simulink model "olamodel"  (Simulink 8.3)
settings: Solver=FixedStepDiscrete  SolverMode=SingleTasking  StartTime=0.0  StopTime=9999999  RelTol=1e-3  AbsTol=1e-6
model workspace (MATLAB code in the model file):
  | olademo
values from neighbouring files (symbols this model uses):
  Fs = AR.SampleRate    [GenDSPTestbenchExample.m]    (also in HelperAircraftKalmanFilter.m = 1000; HelperAudioEqualization.m = 44100; HelperAudioEqualizationCodeGeneration.m = 44100; HelperAudioToneRemoval.m = 44100)
undefined symbols (not defined in the file or in its folder): bitrevorder, ymax, ymin
libraries: dspmathops x3, dspxfrm3 x2, dspsrcs4 x1, dspsigops x1, dspmisc x1, simulink x1
settings Model: Creator=The MathWorks Inc.  CovMetricSettings=d  ExtModeTrigMode=oneshot  ExtModeArmWhenConnect=off
settings DataIOCC: LimitDataPoints=off  SaveOutput=off  SaveTime=off  SignalLoggingName=logsOut
settings OptimizationCC: BlockReduction=off  BooleanDataType=off  ExpressionDepthLimit=2147483647  RollThreshold=2  InitFltsAndDblsToZero=on  EfficientMapNaN2IntZero=off
settings DebuggingCC: SaveWithParameterizedLinksMsg=none  SignalResolutionControl=TryResolveAllWithWarning  SolverPrmCheckMsg=none  MultiTaskDSMMsg=warning  MultiTaskCondExecSysMsg=none  IntegerOverflowMsg=none  FcnCallInpInsideContextMsg=UseLocalSettings  StrictBusMsg=None
settings HardwareCC: ProdHWDeviceType=Specified
settings RTWCC: IncludeERTFirstTime=on
settings GRTTargetCC: TargetFcnLib=ansi_tfl_tmw.mat

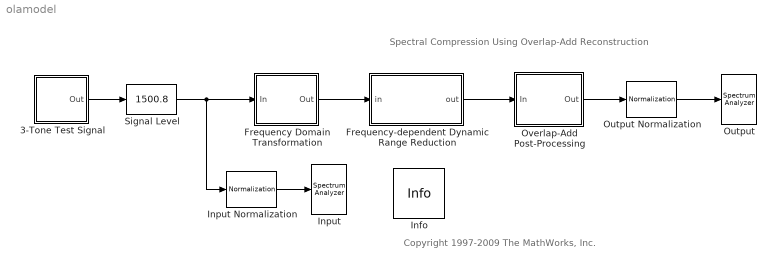
== system olamodel ==
  note: Spectral Compression
      | Using Overlap-Add Reconstruction
  note: Copyright 1997-2009 The MathWorks, Inc.
  3-Tone Test Signal : Subsystem
  Frequency Domain Transformation : Subsystem
  Frequency-dependent Dynamic Range Reduction : Subsystem  mask(Complex Compression){}
      mask Display: disp('Frequency\n\nCompression');
  Info : dspmisc/Info  SystemSampleTime=-1
  Input : SpectrumAnalyzer  ScopeSpecification=DataTag0
  Input Normalization : dspmathops/Normalization  NormType=2-norm  Bias=1e-10  NormOver=Each column  ColComp=on  Dimension=1  outputDataTypeStr=Inherit: Same as accumulator  outputLastDataTypeStr=Inherit: Same as accumulator  outputMin=[]  outputMax=[]  accumDataTypeStr=Inherit: Same as product output  accumLastDataTypeStr=Inherit: Same as product output  roundingMode=Floor  overflowMode=off
  Output : SpectrumAnalyzer  ScopeSpecification=DataTag1
  Output Normalization : dspmathops/Normalization  NormType=2-norm  Bias=1e-10  NormOver=Each column  ColComp=on  Dimension=1  outputDataTypeStr=Inherit: Same as accumulator  outputLastDataTypeStr=Inherit: Same as accumulator  outputMin=[]  outputMax=[]  accumDataTypeStr=Inherit: Same as product output  accumLastDataTypeStr=Inherit: Same as product output  roundingMode=Floor  overflowMode=off
  Overlap-Add Post-Processing : Subsystem
  Signal Level : simulink/Math Operations/Slider Gain  low=1  gain=1500.8  high=7500
  wires:
  Frequency Domain Transformation/1(Out) -> Frequency-dependent Dynamic Range Reduction/1(in)
  Frequency-dependent Dynamic Range Reduction/1(out) -> Overlap-Add Post-Processing/1(In)
  3-Tone Test Signal/1(Out) -> Signal Level/1
  Input Normalization/1 -> Input/1
  Output Normalization/1 -> Output/1
  Overlap-Add Post-Processing/1(Out) -> Output Normalization/1
  Signal Level/1 -> Input Normalization/1, Frequency Domain Transformation/1(In)

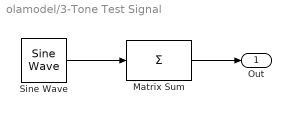
== system olamodel/3-Tone Test Signal ==
  Matrix Sum : Sum  Inputs=+  CollapseMode=Specified dimension  CollapseDim=2  OutDataTypeStr=Inherit: Same as first input
  Sine Wave : dspsrcs4/Sine Wave  Amplitude=1  Frequency=[1024 2048 3072]  Phase=0  SampleMode=Discrete  OutComplex=Real  CompMethod=Trigonometric fcn  TableSize=Speed  SampleTime=1/Fs  SamplesPerFrame=64  ResetState=Restart at time zero  dataType=double  wordLen=16  udDataType=sfix(16)  fracBitsMode=Best precision  numFracBits=15  OutDataTypeStr=double  LastOutDataTypeStr=double
  Out : Outport
  wires:
  Sine Wave/1 -> Matrix Sum/1
  Matrix Sum/1 -> Out/1

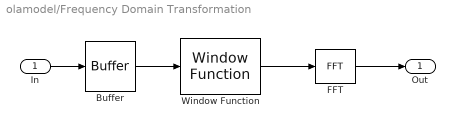
== system olamodel/Frequency Domain Transformation ==
  In : Inport
  Buffer : Buffer  N=256  V=192  TreatMby1Signals=One channel
  FFT : dspxfrm3/FFT  CompMethod=Table lookup  TableOpt=NEW  TableOptActive=Speed  BitRevOrder=on  InheritFFTLength=on  FFTLength=64  WrapInput=on  RowConvenienceOn=on  FFTImplementation=Auto  SkipNorm=off  firstCoeffMode=Specify word length  firstCoeffWordLength=16  firstCoeffFracLength=15  firstCoeffDataTypeStr=fixdt(1,16)  firstCoeffLastDataTypeStr=fixdt(1,16)  outputMin=[]  outputMax=[]  accumDataTypeStr=Inherit: Same as product output  accumLastDataTypeStr=Inherit: Same as product output  roundingMode=Floor  overflowMode=off
  Window Function : dspsigops/Window Function  winmode=Apply window to input  wintype=Hamming  sampmode=Continuous  samptime=1  N=64  Rs=50  beta=10  winsamp=Symmetric  UserWindow=hamming  OptParams=off  UserParams={1.0}  RowConvenienceOn=on  dataType=double  isSigned=on  wordLen=16  udDataType=sfix(16)  fracBitsMode=Best precision  numFracBits=15  roundingMode=Floor  overflowMode=off  numSidelobes=4  sidelobeLevel=-30
  Out : Outport
  wires:
  Buffer/1 -> Window Function/1
  Window Function/1 -> FFT/1
  In/1 -> Buffer/1
  FFT/1 -> Out/1

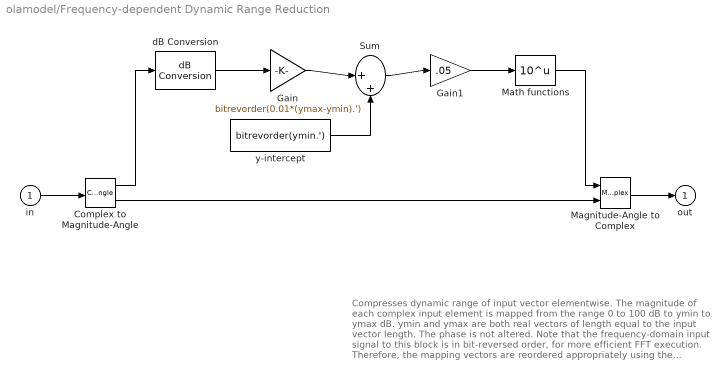
== system olamodel/Frequency-dependent Dynamic Range Reduction ==
  note: Compresses dynamic range of input vector elementwise.
      |
      |  The magnitude of each complex input element is mapped from the range
      |  0 to 100 dB to ymin to ymax dB. ymin and ymax are both real vectors
      | of length equal to the input vector length.  The phase is not altered.
      |
      | Note that the frequency-domain input signal to this block is in
      | bit-reversed order, for more efficient FFT execution.  Therefore, the
      | mapping vectors are reordered appropriately using the "bitrevorder"
      | function in the constant and gain block parameters above.
  in : Inport
  Complex to Magnitude-Angle : ComplexToMagnitudeAngle
  Gain : Gain  Gain=bitrevorder(0.01*(ymax-ymin).')  SaturateOnIntegerOverflow=on  OutDataTypeStr=Inherit: Same as input  ParamDataTypeStr=Inherit: Same as input
  Gain1 : Gain  Gain=.05  SaturateOnIntegerOverflow=on  OutDataTypeStr=Inherit: Same as input  ParamDataTypeStr=Inherit: Same as input
  Magnitude-Angle to Complex : MagnitudeAngleToComplex
  Math functions : Math  Operator=10^u  SaturateOnIntegerOverflow=on
  Sum : Sum  Inputs=|++  SaturateOnIntegerOverflow=on  InputSameDT=on  OutDataTypeStr=Inherit: Same as first input
  dB Conversion : dspmathops/dB Conversion  dBtype=dB  intype=Amplitude  R=1  fuzz=on
  y-intercept : Constant  Value=bitrevorder(ymin.')  VectorParams1D=off
  out : Outport
  wires:
  Complex to Magnitude-Angle/2 -> Magnitude-Angle to Complex/2
  in/1 -> Complex to Magnitude-Angle/1
  Magnitude-Angle to Complex/1 -> out/1
  dB Conversion/1 -> Gain/1
  Gain/1 -> Sum/1
  Sum/1 -> Gain1/1
  y-intercept/1 -> Sum/2
  Gain1/1 -> Math functions/1
  Complex to Magnitude-Angle/1 -> dB Conversion/1
  Math functions/1 -> Magnitude-Angle to Complex/1

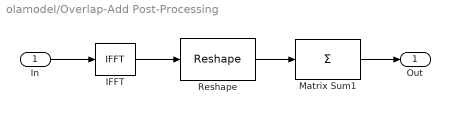
== system olamodel/Overlap-Add Post-Processing ==
  In : Inport
  IFFT : dspxfrm3/IFFT  CompMethod=Table lookup  TableOpt=HYBRID  TableOptActive=Speed  BitRevOrder=on  cs_in=on  SkipNorm=on  InheritFFTLength=on  FFTLength=64  WrapInput=on  mode=Real  outSamplingMode=Frame based  RowConvenienceOn=on  FFTImplementation=Auto  firstCoeffMode=Specify word length  firstCoeffWordLength=16  firstCoeffFracLength=15  firstCoeffDataTypeStr=fixdt(1,16)  firstCoeffLastDataTypeStr=fixdt(1,16)  outputMin=[]  outputMax=[]  accumDataTypeStr=Inherit: Same as product output  accumLastDataTypeStr=Inherit: Same as product output  roundingMode=Floor  overflowMode=off
  Matrix Sum1 : Sum  Inputs=+  CollapseMode=Specified dimension  CollapseDim=2  OutDataTypeStr=Inherit: Same as first input
  Reshape : Reshape  OutputDimensionality=Customize  OutputDimensions=[64 4]
  Out : Outport
  wires:
  Reshape/1 -> Matrix Sum1/1
  IFFT/1 -> Reshape/1
  Matrix Sum1/1 -> Out/1
  In/1 -> IFFT/1
